simulink model "new_ipc_control1"  (Simulink 7.1)
settings: Solver=ode3  StartTime=0.0  StopTime=120  FixedStep=0.01  RelTol=1e-3
values from neighbouring files (symbols this model uses):
  C = abs(d-B)    [fuzzycontrol.m]    (also in lv_demofile6.m = 1450000)
  Jem = 90    [lv_cankaofile.m]    (also in lv_demofile.m = 97.5; lv_demofile1.m = 97.5; lv_demofile2.m = 97.5; lv_demofile3.m = 97.5)
  Jwt = 9e7    (= 90000000)    [lv_cankaofile.m]    (also in lv_demofile.m = 3275300; lv_demofile1.m = 3275300; lv_demofile2.m = 3275300; lv_demofile3.m = 3275300)
  K = 83    [lv_cankaofile.m]    (also in lv_demofile.m; lv_demofile1.m = 75.76; lv_demofile2.m; lv_demofile3.m = 75.76)
  R = 40    [lv_cankaofile.m]    (also in lv_demofile.m = 38.5; lv_demofile1.m = 38.75; lv_demofile2.m = 38.5; lv_demofile3.m = 38.5)
  ro_air = 1.225    [lv_cankaofile.m]    (also in lv_demofile.m = 1.2236; lv_demofile1.m; lv_demofile2.m = 1.2236; lv_demofile3.m)
undefined symbols (not defined in the file or in its folder): xishu
libraries: wt_blockset_v3 x4, simulink_extras x1, DRlib x1
settings Model: Creator=lv  LastModifiedBy=lv

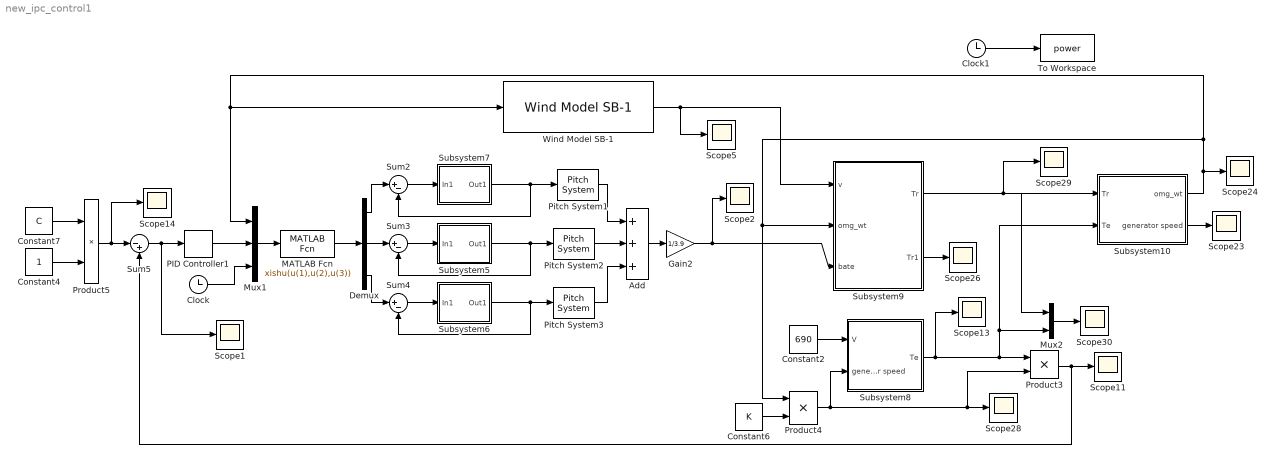
== system new_ipc_control1 ==
  Add : Sum  Inputs=+++  OutDataType=sfix(16)  OutScaling=2^-10
  Clock : Clock
      settings: Decimation=10
  Clock1 : Clock
      settings: Decimation=10
  Constant2 : Constant  Value=690  OutDataType=sfix(16)  OutScaling=2^0
  Constant4 : Constant  OutDataType=sfix(16)  OutScaling=2^0
  Constant6 : Constant  Value=K  OutDataType=sfix(16)  OutScaling=2^0
  Constant7 : Constant  Value=C  OutDataType=sfix(16)  OutScaling=2^0
  Demux : Demux  Outputs=3
  Gain2 : Gain  Gain=1/3.9  ParameterDataType=sfix(16)  ParameterScaling=2^0  OutDataType=sfix(16)  OutScaling=2^0
  MATLAB Fcn : MATLABFcn  MATLABFcn=xishu(u(1),u(2),u(3))
  Mux1 : Mux  Inputs=3
  Mux2 : Mux  Inputs=2
  PID Controller1 : simulink_extras/Additional Linear/PID Controller  SystemSampleTime=-1  P=16.415  I=0.005  D=2
  Pitch System1 : wt_blockset_v3/Control/WT Controller 2 MW DFIG/Pitch System  SystemSampleTime=-1
      link override Saturation1: LowerLimit=-90
  Pitch System2 : wt_blockset_v3/Control/WT Controller 2 MW DFIG/Pitch System  SystemSampleTime=-1
      link override Saturation1: LowerLimit=-90
  Pitch System3 : wt_blockset_v3/Control/WT Controller 2 MW DFIG/Pitch System  SystemSampleTime=-1
      link override Saturation1: LowerLimit=-90
  Product3 : Product  OutDataType=sfix(16)  OutScaling=2^0  RndMeth=Zero
  Product4 : Product  OutDataType=sfix(16)  OutScaling=2^0  RndMeth=Zero
  Product5 : Product  OutDataType=sfix(16)  OutScaling=2^0  RndMeth=Zero
  Scope{1..2,5,11,13..14,23..24,26,28..30} (12 alike) : Scope
      Scope1 settings: YMin=-8000  YMax=9000
      Scope11 settings: TimeRange=100  YMin=1.47e+006  YMax=1.5275e+006  SaveName=ipower2
      Scope13 settings: YMin=3424.13  YMax=3784.57  SaveName=ScopeData29
      Scope14 settings: YMin=-51201.2  YMax=-51201.1  SaveName=ScopeData31
      Scope2 settings: YMin=11  YMax=27  SaveName=ScopeData14
      Scope23 settings: YMin=75.6077  YMax=83.5665  SaveName=ScopeData37
      Scope24 settings: YMin=1.96962  YMax=1.96971  SaveName=ScopeData38
      Scope26 settings: SaveName=ScopeData40
      Scope28 settings: YMin=292.336  YMax=292.336  SaveName=ScopeData41
      Scope29 settings: YMin=725000  YMax=1.025e+006  SaveName=ScopeData42
      Scope30 settings: TimeRange=12  YMin=0  YMax=275000  SaveName=ScopeData43
      Scope5 settings: YMin=2.5  YMax=25  SaveName=ScopeData17
  Subsystem10 : Subsystem
  Subsystem5 : Subsystem
  Subsystem6 : Subsystem
  Subsystem7 : Subsystem
  Subsystem8 : Subsystem
  Subsystem9 : Subsystem
  Sum2 : Sum  Inputs=|+-  OutDataType=sfix(16)  OutScaling=2^0  SaturateOnIntegerOverflow=on
  Sum3 : Sum  Inputs=|+-  OutDataType=sfix(16)  OutScaling=2^0  SaturateOnIntegerOverflow=on
  Sum4 : Sum  Inputs=|+-  OutDataType=sfix(16)  OutScaling=2^0  SaturateOnIntegerOverflow=on
  Sum5 : Sum  Inputs=|-+  OutDataType=sfix(16)  OutScaling=2^0  SaturateOnIntegerOverflow=on
  To Workspace : ToWorkspace  VariableName=power  SampleTime=-1  SaveFormat=Array
  Wind Model SB-1 : wt_blockset_v3/Mechanical Components/Wind Model SB-1  SystemSampleTime=-1  D_rotor=77  v_mean=14  roughness=600  turb_int=12  T_sample=0.01
  wires:
  Subsystem7/1(Out1) -> Sum2/2, Pitch System1/1
  Sum2/1 -> Subsystem7/1(In1)
  Subsystem5/1(Out1) -> Sum3/2, Pitch System2/1
  Sum3/1 -> Subsystem5/1(In1)
  Subsystem6/1(Out1) -> Sum4/2, Pitch System3/1
  Sum4/1 -> Subsystem6/1(In1)
  MATLAB Fcn/1 -> Demux/1
  Demux/2 -> Sum3/1
  Demux/1 -> Sum2/1
  Demux/3 -> Sum4/1
  Mux1/1 -> MATLAB Fcn/1
  PID Controller1/1 -> Mux1/2
  Clock/1 -> Mux1/3
  Pitch System1/1 -> Add/1
  Pitch System2/1 -> Add/2
  Pitch System3/1 -> Add/3
  Add/1 -> Gain2/1
  Subsystem8/1(Te) -> Scope13/1, Subsystem10/2(Te), Mux2/2, Product3/1
  Subsystem10/2(generator speed) -> Scope23/1
  Constant2/1 -> Subsystem8/1(V)
  Subsystem10/1(omg_wt) -> Scope24/1, Subsystem9/2(omg_wt), Product4/1, Mux1/1, Wind Model SB-1/1
  Product3/1 -> Scope11/1, Sum5/2
  Subsystem9/2(Tr1) -> Scope26/1
  Constant6/1 -> Product4/2
  Product4/1 -> Subsystem8/2(generator speed), Product3/2, Scope28/1
  Subsystem9/1(Tr) -> Subsystem10/1(Tr), Scope29/1, Mux2/1
  Mux2/1 -> Scope30/1
  Gain2/1 -> Subsystem9/3(bate), Scope2/1
  Constant7/1 -> Product5/1
  Product5/1 -> Sum5/1, Scope14/1
  Constant4/1 -> Product5/2
  Sum5/1 -> PID Controller1/1, Scope1/1
  Clock1/1 -> To Workspace/1
  Wind Model SB-1/1 -> Subsystem9/1(v), Scope5/1

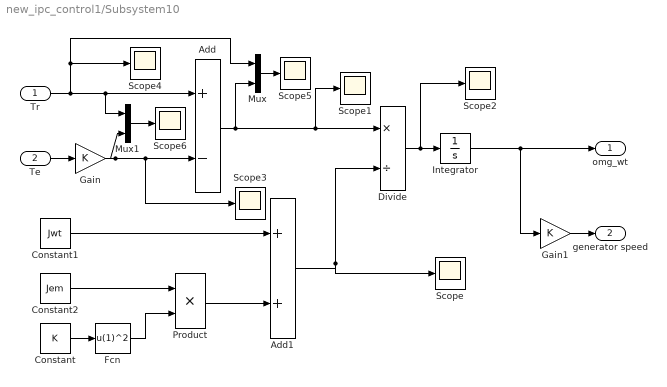
== system new_ipc_control1/Subsystem10 ==
  Tr : Inport  OutDataType=sfix(16)  OutScaling=2^0
  Te : Inport  Port=2  OutDataType=sfix(16)  OutScaling=2^0
  Add : Sum  Inputs=+-  OutDataType=sfix(16)  OutScaling=2^-10
  Add1 : Sum  OutDataType=sfix(16)  OutScaling=2^-10
  Constant : Constant  Value=K  OutDataType=sfix(16)  OutScaling=2^0
  Constant1 : Constant  Value=Jwt  OutDataType=sfix(16)  OutScaling=2^0
  Constant2 : Constant  Value=Jem  OutDataType=sfix(16)  OutScaling=2^0
  Divide : Product  Inputs=*/  OutDataType=sfix(16)  OutScaling=2^-10
  Fcn : Fcn  Expr=u(1)^2
  Gain : Gain  Gain=K  ParameterDataType=sfix(16)  ParameterScaling=2^0  OutDataType=sfix(16)  OutScaling=2^0
  Gain1 : Gain  Gain=K  ParameterDataType=sfix(16)  ParameterScaling=2^0  OutDataType=sfix(16)  OutScaling=2^0
  Integrator : Integrator  InitialCondition=1.96885526
  Mux : Mux  Inputs=2
  Mux1 : Mux  Inputs=2
  Product : Product  OutDataType=sfix(16)  OutScaling=2^0  RndMeth=Zero
  Scope{,1..6} (7 alike) : Scope
      Scope settings: SaveName=ScopeData5
      Scope1 settings: YMin=1.3446e-008  YMax=1.3446e-008  SaveName=ScopeData6
      Scope2 settings: SaveName=ScopeData7
      Scope3 settings: SaveName=ScopeData23
      Scope4 settings: SaveName=ScopeData24
      Scope5 settings: SaveName=ScopeData25
      Scope6 settings: YMin=326577  YMax=326577  SaveName=ScopeData3
  omg_wt : Outport  OutDataType=sfix(16)  OutScaling=2^0
  generator speed : Outport  Port=2  OutDataType=sfix(16)  OutScaling=2^0
  wires:
  Fcn/1 -> Product/2
  Constant/1 -> Fcn/1
  Te/1 -> Gain/1
  Tr/1 -> Scope4/1, Mux/1, Add/1, Mux1/1
  Gain/1 -> Add/2, Scope3/1, Mux1/2
  Constant2/1 -> Product/1
  Constant1/1 -> Add1/1
  Product/1 -> Add1/2
  Add/1 -> Scope1/1, Divide/1, Mux/2
  Add1/1 -> Scope/1, Divide/2
  Divide/1 -> Scope2/1, Integrator/1
  Integrator/1 -> Gain1/1, omg_wt/1
  Gain1/1 -> generator speed/1
  Mux/1 -> Scope5/1
  Mux1/1 -> Scope6/1

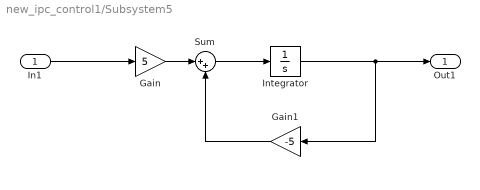
== system new_ipc_control1/Subsystem5 ==
  In1 : Inport  OutDataType=sfix(16)  OutScaling=2^0
  Gain : Gain  Gain=5  ParameterDataType=sfix(16)  ParameterScaling=2^0  OutDataType=sfix(16)  OutScaling=2^0
  Gain1 : Gain  Orientation=left  Gain=-5  ParameterDataType=sfix(16)  ParameterScaling=2^0  OutDataType=sfix(16)  OutScaling=2^0
  Integrator : Integrator
  Sum : Sum  Inputs=|++  OutDataType=sfix(16)  OutScaling=2^0
  Out1 : Outport  OutDataType=sfix(16)  OutScaling=2^0
  wires:
  Integrator/1 -> Gain1/1, Out1/1
  Gain1/1 -> Sum/2
  Sum/1 -> Integrator/1
  Gain/1 -> Sum/1
  In1/1 -> Gain/1

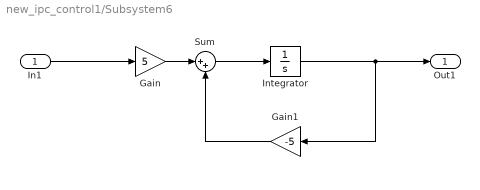
== system new_ipc_control1/Subsystem6 ==
  In1 : Inport  OutDataType=sfix(16)  OutScaling=2^0
  Gain : Gain  Gain=5  ParameterDataType=sfix(16)  ParameterScaling=2^0  OutDataType=sfix(16)  OutScaling=2^0
  Gain1 : Gain  Orientation=left  Gain=-5  ParameterDataType=sfix(16)  ParameterScaling=2^0  OutDataType=sfix(16)  OutScaling=2^0
  Integrator : Integrator
  Sum : Sum  Inputs=|++  OutDataType=sfix(16)  OutScaling=2^0
  Out1 : Outport  OutDataType=sfix(16)  OutScaling=2^0
  wires:
  Integrator/1 -> Gain1/1, Out1/1
  Gain1/1 -> Sum/2
  Sum/1 -> Integrator/1
  Gain/1 -> Sum/1
  In1/1 -> Gain/1

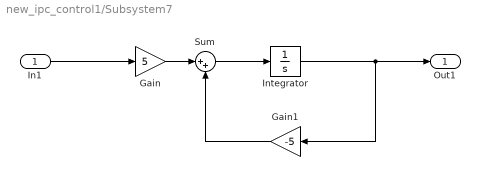
== system new_ipc_control1/Subsystem7 ==
  In1 : Inport  OutDataType=sfix(16)  OutScaling=2^0
  Gain : Gain  Gain=5  ParameterDataType=sfix(16)  ParameterScaling=2^0  OutDataType=sfix(16)  OutScaling=2^0
  Gain1 : Gain  Orientation=left  Gain=-5  ParameterDataType=sfix(16)  ParameterScaling=2^0  OutDataType=sfix(16)  OutScaling=2^0
  Integrator : Integrator
  Sum : Sum  Inputs=|++  OutDataType=sfix(16)  OutScaling=2^0
  Out1 : Outport  OutDataType=sfix(16)  OutScaling=2^0
  wires:
  Integrator/1 -> Gain1/1, Out1/1
  Gain1/1 -> Sum/2
  Sum/1 -> Integrator/1
  Gain/1 -> Sum/1
  In1/1 -> Gain/1

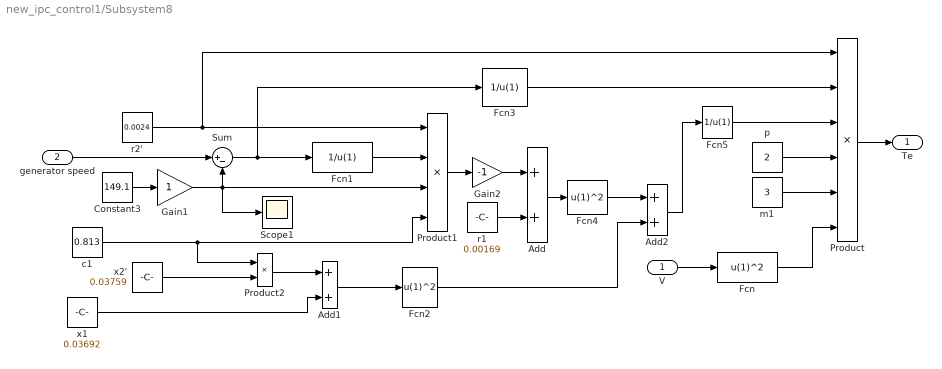
== system new_ipc_control1/Subsystem8 ==
  V : Inport  OutDataType=sfix(16)  OutScaling=2^0
  generator speed : Inport  Port=2  OutDataType=sfix(16)  OutScaling=2^0
  Add : Sum  OutDataType=sfix(16)  OutScaling=2^-10
  Add1 : Sum  OutDataType=sfix(16)  OutScaling=2^-10
  Add2 : Sum  OutDataType=sfix(16)  OutScaling=2^-10
  Constant3 : Constant  Value=149.1  OutDataType=sfix(16)  OutScaling=2^0
  Fcn : Fcn  Expr=u(1)^2
  Fcn1 : Fcn  Expr=1/u(1)
  Fcn2 : Fcn  Expr=u(1)^2
  Fcn3 : Fcn  Expr=1/u(1)
  Fcn4 : Fcn  Expr=u(1)^2
  Fcn5 : Fcn  Expr=1/u(1)
  Gain1 : Gain  ParameterDataType=sfix(16)  ParameterScaling=2^0  OutDataType=sfix(16)  OutScaling=2^0
  Gain2 : Gain  Gain=-1  ParameterDataType=sfix(16)  ParameterScaling=2^0  OutDataType=sfix(16)  OutScaling=2^0
  Product : Product  Inputs=6  OutDataType=sfix(16)  OutScaling=2^0  RndMeth=Zero
  Product1 : Product  Inputs=4  OutDataType=sfix(16)  OutScaling=2^0  RndMeth=Zero
  Product2 : Product  OutDataType=sfix(16)  OutScaling=2^0  RndMeth=Zero
  Scope1 : Scope
      settings: SaveName=ScopeData10
  Sum : Sum  Inputs=|+-  OutDataType=sfix(16)  OutScaling=2^0
  c1 : Constant  Value=0.813  OutDataType=sfix(16)  OutScaling=2^0
  m1 : Constant  Value=3  OutDataType=sfix(16)  OutScaling=2^0
  p : Constant  Value=2  OutDataType=sfix(16)  OutScaling=2^0
  r1 : Constant  Value=0.00169  OutDataType=sfix(16)  OutScaling=2^0
  r2' : Constant  Value=0.0024  OutDataType=sfix(16)  OutScaling=2^0
  x1 : Constant  Value=0.03692  OutDataType=sfix(16)  OutScaling=2^0
  x2' : Constant  Value=0.03759  OutDataType=sfix(16)  OutScaling=2^0
  Te : Outport  OutDataType=sfix(16)  OutScaling=2^0
  wires:
  V/1 -> Fcn/1
  generator speed/1 -> Sum/1
  Constant3/1 -> Gain1/1
  Gain1/1 -> Sum/2, Product1/3, Scope1/1
  Sum/1 -> Fcn3/1, Fcn1/1
  r2'/1 -> Product1/1, Product/1
  Fcn1/1 -> Product1/2
  c1/1 -> Product1/4, Product2/1
  x2'/1 -> Product2/2
  Product2/1 -> Add1/1
  x1/1 -> Add1/2
  Add1/1 -> Fcn2/1
  Product1/1 -> Gain2/1
  r1/1 -> Add/2
  Gain2/1 -> Add/1
  Add/1 -> Fcn4/1
  Fcn4/1 -> Add2/1
  Fcn2/1 -> Add2/2
  Add2/1 -> Fcn5/1
  Product/1 -> Te/1
  Fcn3/1 -> Product/2
  Fcn5/1 -> Product/3
  p/1 -> Product/4
  m1/1 -> Product/5
  Fcn/1 -> Product/6

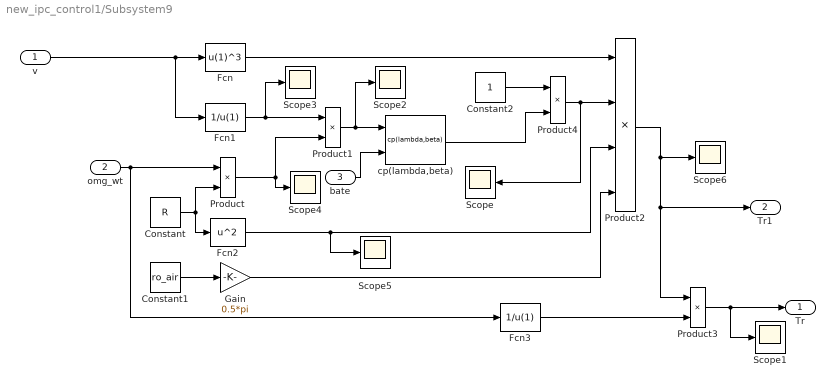
== system new_ipc_control1/Subsystem9 ==
  v : Inport  OutDataType=sfix(16)  OutScaling=2^0
  omg_wt : Inport  Port=2  OutDataType=sfix(16)  OutScaling=2^0
  bate : Inport  Port=3  OutDataType=sfix(16)  OutScaling=2^0
  Constant : Constant  Value=R  OutDataType=sfix(16)  OutScaling=2^0
  Constant1 : Constant  Value=ro_air  OutDataType=sfix(16)  OutScaling=2^0
  Constant2 : Constant  OutDataType=sfix(16)  OutScaling=2^0
  Fcn : Fcn  Expr=u(1)^3
  Fcn1 : Fcn  Expr=1/u(1)
  Fcn2 : Fcn  Expr=u^2
  Fcn3 : Fcn  Expr=1/u(1)
  Gain : Gain  Gain=0.5*pi  ParameterDataType=sfix(16)  ParameterScaling=2^0  OutDataType=sfix(16)  OutScaling=2^0
  Product{,1,3..4} (4 alike) : Product  OutDataType=sfix(16)  OutScaling=2^0  RndMeth=Zero
  Product2 : Product  Inputs=4  OutDataType=sfix(16)  OutScaling=2^0  RndMeth=Zero
  Scope{,1..6} (7 alike) : Scope
      Scope settings: TimeRange=50  YMin=0.1772981595092024  YMax=0.2028981595092024  SaveName=ScopeData4
      Scope1 settings: TimeRange=20  YMin=-1500000  YMax=1500000
      Scope2 settings: SaveName=ScopeData6
      Scope3 settings: SaveName=ScopeData7
      Scope4 settings: SaveName=ScopeData8
      Scope5 settings: YMin=1426.48  YMax=1576.64  SaveName=ScopeData20
      Scope6 settings: TimeRange=20  YMin=-500000  YMax=5e+006  SaveName=ScopeData21
  cp(lambda,beta) : DRlib/Wind Generation/Wind Turbine/cp(lambda,beta)  SystemSampleTime=-1
  Tr : Outport  OutDataType=sfix(16)  OutScaling=2^0
  Tr1 : Outport  Port=2  OutDataType=sfix(16)  OutScaling=2^0
  wires:
  v/1 -> Fcn/1, Fcn1/1
  omg_wt/1 -> Product/1, Fcn3/1
  Constant/1 -> Product/2, Fcn2/1
  Fcn1/1 -> Product1/1, Scope3/1
  Product/1 -> Product1/2, Scope4/1
  Product1/1 -> Scope2/1, cp(lambda,beta)/1
  bate/1 -> cp(lambda,beta)/2
  Fcn/1 -> Product2/1
  cp(lambda,beta)/1 -> Product4/2
  Fcn2/1 -> Product2/3, Scope5/1
  Gain/1 -> Product2/4
  Constant1/1 -> Gain/1
  Product2/1 -> Scope6/1, Product3/1, Tr1/1
  Fcn3/1 -> Product3/2
  Product3/1 -> Scope1/1, Tr/1
  Product4/1 -> Product2/2, Scope/1
  Constant2/1 -> Product4/1
